simulink model "simulationModel"  (R2022b)
settings: Solver=VariableStepAuto  StartTime=0.0  StopTime=20.0  MaxStep=2e-3  RelTol=1e-3
values from neighbouring files (symbols this model uses):
  k = 1e-6    (= 1e-06)    [simulation.m]
  K_c_PI1 = 0.15/k+(0.35-(theta*tau)/(theta+tau)^2)*(tau/(k*theta))    (= 1899030.33908)    [simulation.m]
  K_c_PI2 = 1/k*(tau/(tau/3+theta))    (= 2117647.05882)    [simulation.m]
  K_c_PID1 = 1/k*(0.2+0.45*(tau/theta))    (= 3440000)    [simulation.m]
  K_c_PID2 = 1/k*(2*tau+theta)/(2*tau/3+theta)    (= 2655172.41379)    [simulation.m]
  tau = 1.8    [simulation.m]
  tau_d_PID1 = (0.5*theta*tau)/(0.3*theta+tau)    (= 0.12)    [simulation.m]
  tau_d_PID2 = (tau*theta)/(2*tau+theta)    (= 0.116883116883)    [simulation.m]
  tau_i_PI1 = 0.35*theta+(13*theta*tau^2)/(tau^2+12*theta*tau+7*theta^2)    (= 1.24751101625)    [simulation.m]
  tau_i_PI2 = tau    (= 1.8)    [simulation.m]
  tau_i_PID1 = theta*(0.4*theta+0.8*tau)/(theta+0.1*tau)    (= 0.895348837209)    [simulation.m]
  tau_i_PID2 = tau+theta/2    (= 1.925)    [simulation.m]
  theta = 0.25    [simulation.m]
settings Model: Creator=omare  LastModifiedBy=omare
settings DataIOCC: ReturnWorkspaceOutputs=off

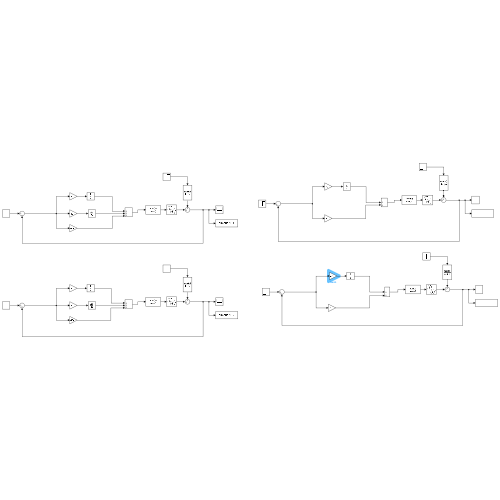
[thumbnail: Simulink's stored preview of the top-level diagram]
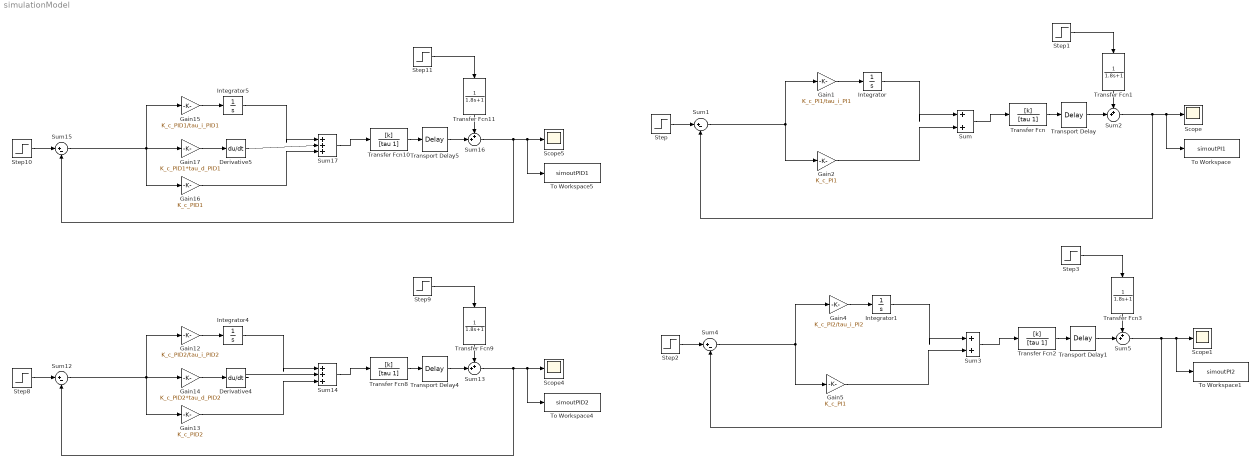
== system simulationModel ==
  Derivative4 : Derivative
  Derivative5 : Derivative
  Gain1 : Gain  Gain=K_c_PI1/tau_i_PI1
  Gain12 : Gain  Gain=K_c_PID2/tau_i_PID2
  Gain13 : Gain  Gain=K_c_PID2
  Gain14 : Gain  Gain=K_c_PID2*tau_d_PID2
  Gain15 : Gain  Gain=K_c_PID1/tau_i_PID1
  Gain16 : Gain  Gain=K_c_PID1
  Gain17 : Gain  Gain=K_c_PID1*tau_d_PID1
  Gain2 : Gain  Gain=K_c_PI1
  Gain4 : Gain  Gain=K_c_PI2/tau_i_PI2
  Gain5 : Gain  Gain=K_c_PI1
  Integrator{,1,4..5} (4 alike) : Integrator
  Scope{,1,4..5} (4 alike) : Scope
  Step{,2,8,10} (4 alike) : Step  Time=0  SampleTime=0
  Step{1,3,9,11} (4 alike) : Step  Time=12  After=0  SampleTime=0
  Sum : Sum  Inputs=|++
  Sum{1,4,12,15} (4 alike) : Sum  Inputs=|+-
  Sum{2,5,13,16} (4 alike) : Sum  Inputs=++|
  Sum14 : Sum  Inputs=|+++
  Sum17 : Sum  Inputs=|+++
  Sum3 : Sum  Inputs=|++
  To Workspace : ToWorkspace  VariableName=simoutPI1  SaveFormat=Timeseries  SampleTime=-1
  To Workspace1 : ToWorkspace  VariableName=simoutPI2  SaveFormat=Timeseries  SampleTime=-1
  To Workspace4 : ToWorkspace  VariableName=simoutPID2  SaveFormat=Timeseries  SampleTime=-1
  To Workspace5 : ToWorkspace  VariableName=simoutPID1  SaveFormat=Timeseries  SampleTime=-1
  Transfer Fcn{,2,8,10} (4 alike) : TransferFcn  Numerator=[k]  Denominator=[tau 1]
  Transfer Fcn{1,3,9,11} (4 alike) : TransferFcn  Denominator=[1.8 1]
  Transport Delay{,1,4..5} (4 alike) : TransportDelay  DelayTime=theta
  wires:
  Gain1/1 -> Integrator/1
  Integrator/1 -> Sum/1
  Gain2/1 -> Sum/2
  Sum/1 -> Transfer Fcn/1
  Transfer Fcn/1 -> Transport Delay/1
  Step/1 -> Sum1/1
  Sum1/1 -> Gain1/1, Gain2/1
  Sum2/1 -> To Workspace/1, Scope/1, Sum1/2
  Transport Delay/1 -> Sum2/2
  Transfer Fcn1/1 -> Sum2/1
  Step1/1 -> Transfer Fcn1/1
  Sum5/1 -> To Workspace1/1, Scope1/1, Sum4/2
  Transfer Fcn3/1 -> Sum5/1
  Step3/1 -> Transfer Fcn3/1
  Transport Delay1/1 -> Sum5/2
  Transfer Fcn2/1 -> Transport Delay1/1
  Sum3/1 -> Transfer Fcn2/1
  Gain4/1 -> Integrator1/1
  Integrator1/1 -> Sum3/1
  Sum4/1 -> Gain5/1, Gain4/1
  Step2/1 -> Sum4/1
  Sum17/1 -> Transfer Fcn10/1
  Gain16/1 -> Sum17/3
  Sum16/1 -> To Workspace5/1, Scope5/1, Sum15/2
  Transport Delay5/1 -> Sum16/2
  Gain15/1 -> Integrator5/1
  Derivative5/1 -> Sum17/2
  Step11/1 -> Transfer Fcn11/1
  Transfer Fcn11/1 -> Sum16/1
  Sum15/1 -> Gain15/1, Gain16/1, Gain17/1
  Step10/1 -> Sum15/1
  Integrator5/1 -> Sum17/1
  Transfer Fcn10/1 -> Transport Delay5/1
  Gain17/1 -> Derivative5/1
  Integrator4/1 -> Sum14/1
  Gain14/1 -> Derivative4/1
  Sum12/1 -> Gain12/1, Gain13/1, Gain14/1
  Step8/1 -> Sum12/1
  Transfer Fcn9/1 -> Sum13/1
  Step9/1 -> Transfer Fcn9/1
  Derivative4/1 -> Sum14/2
  Gain12/1 -> Integrator4/1
  Transport Delay4/1 -> Sum13/2
  Transfer Fcn8/1 -> Transport Delay4/1
  Gain13/1 -> Sum14/3
  Sum14/1 -> Transfer Fcn8/1
  Sum13/1 -> To Workspace4/1, Scope4/1, Sum12/2
  Gain5/1 -> Sum3/2
